simulink model "DistrictRolloutModel"  (R2026a)
settings: Solver=VariableStepAuto
settings Model: Creator=sneha  LastModifiedBy=sneha

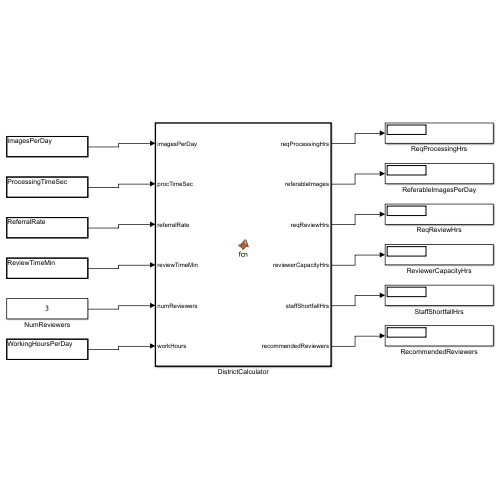
[thumbnail: Simulink's stored preview of the top-level diagram]
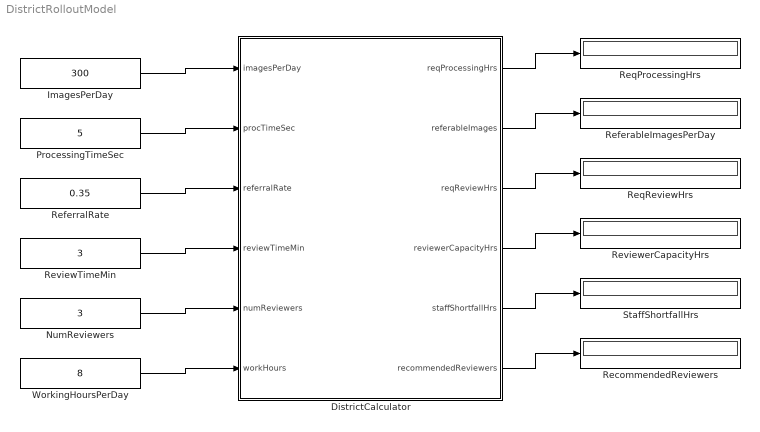
== system DistrictRolloutModel ==
  DistrictCalculator : MATLAB Function  TreatAsAtomicUnit=on
  ImagesPerDay : Constant  Value=300
  NumReviewers : Constant  Value=3
  ProcessingTimeSec : Constant  Value=5
  RecommendedReviewers : Display
  ReferableImagesPerDay : Display
  ReferralRate : Constant  Value=0.35
  ReqProcessingHrs : Display
  ReqReviewHrs : Display
  ReviewTimeMin : Constant  Value=3
  ReviewerCapacityHrs : Display
  StaffShortfallHrs : Display
  WorkingHoursPerDay : Constant  Value=8
  wires:
  ImagesPerDay/1 -> DistrictCalculator/1(imagesPerDay)
  ProcessingTimeSec/1 -> DistrictCalculator/2(procTimeSec)
  ReferralRate/1 -> DistrictCalculator/3(referralRate)
  ReviewTimeMin/1 -> DistrictCalculator/4(reviewTimeMin)
  NumReviewers/1 -> DistrictCalculator/5(numReviewers)
  WorkingHoursPerDay/1 -> DistrictCalculator/6(workHours)
  DistrictCalculator/1(reqProcessingHrs) -> ReqProcessingHrs/1
  DistrictCalculator/2(referableImages) -> ReferableImagesPerDay/1
  DistrictCalculator/3(reqReviewHrs) -> ReqReviewHrs/1
  DistrictCalculator/4(reviewerCapacityHrs) -> ReviewerCapacityHrs/1
  DistrictCalculator/5(staffShortfallHrs) -> StaffShortfallHrs/1
  DistrictCalculator/6(recommendedReviewers) -> RecommendedReviewers/1

== matlab function DistrictRolloutModel/DistrictCalculator ==
  data: imagesPerDay input; reqProcessingHrs output; procTimeSec input; referralRate input; reviewTimeMin input; numReviewers input; workHours input; referableImages output; reqReviewHrs output; reviewerCapacityHrs output; staffShortfallHrs output; recommendedReviewers output
function [reqProcessingHrs, referableImages, reqReviewHrs, reviewerCapacityHrs, staffShortfallHrs, recommendedReviewers] = districtCalc(imagesPerDay, procTimeSec, referralRate, reviewTimeMin, numReviewers, workHours)
% Hours of AI processing time needed per day
reqProcessingHrs = imagesPerDay * procTimeSec / 3600;

% How many of those images actually need a human doctor to look
referableImages = imagesPerDay * referralRate;

% Hours of doctor review time needed per day
reqReviewHrs = referableImages * reviewTimeMin / 60;

% Hours of review capacity the current staff actually provides
reviewerCapacityHrs = numReviewers * workHours;

% If required > available, this is how many hours short you are
staffShortfallHrs = max(0, reqReviewHrs - reviewerCapacityHrs);

% How many reviewers you would actually need to keep up
recommendedReviewers = ceil(reqReviewHrs / workHours);
end
